simulink model "mppt_top"  (R2025b)
settings: Solver=FixedStepAuto  StartTime=0.0  StopTime=0.05  RelTol=1e-3
PreLoadFcn:
  | addpath('C:\Users\PRANAV\Downloads\ResearchWorks\hdlimport\mppt_top');
libraries: fl_lib x10, simulink x9, nesl_utility x6, hdlsllib x4, ee_lib x1
CloseFcn:
  | addpath('C:\Users\PRANAV\Downloads\ResearchWorks\hdlimport\mppt_top');
  | rmpath('C:\Users\PRANAV\Downloads\ResearchWorks\hdlimport\mppt_top');
settings Model: DataTypeOverride=Off  Creator=PRANAV  LastModifiedBy=PRANAV
settings OptimizationCC: BlockReduction=off  ConditionallyExecuteInputs=off  DefaultParameterBehavior=Inlined  InheritOutputTypeSmallerThanSingle=on
settings DebuggingCC: ArtificialAlgebraicLoopMsg=error  InheritedTsInSrcMsg=none  SingleTaskRateTransMsg=error
settings HardwareCC: ProdBitPerPointer=32.0  ProdBitPerSizeT=32.0  ProdBitPerPtrDiffT=32.0  ProdLargestAtomicFloat=None  ProdIntDivRoundTo=Undefined  ProdEndianess=Unspecified  ProdWordSize=32.0  ProdHWDeviceType=ASIC/FPGA->ASIC/FPGA  TargetBitPerPointer=64.0  TargetBitPerSizeT=64.0  TargetBitPerPtrDiffT=64.0  TargetLongLongMode=on  TargetIntDivRoundTo=Zero  TargetEndianess=LittleEndian  TargetWordSize=64.0  TargetHWDeviceType=Custom Processor->MATLAB Host Computer  ProdEqTarget=off

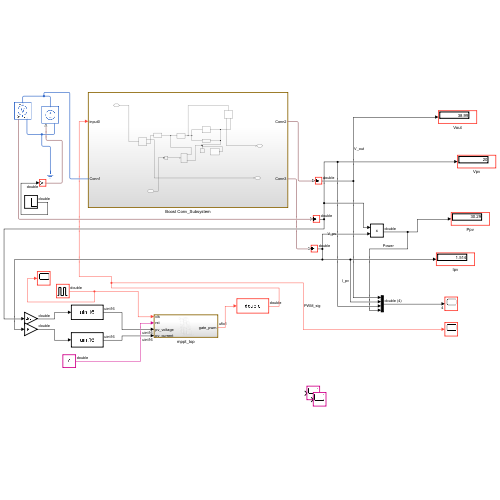
[thumbnail: Simulink's stored preview of the top-level diagram]
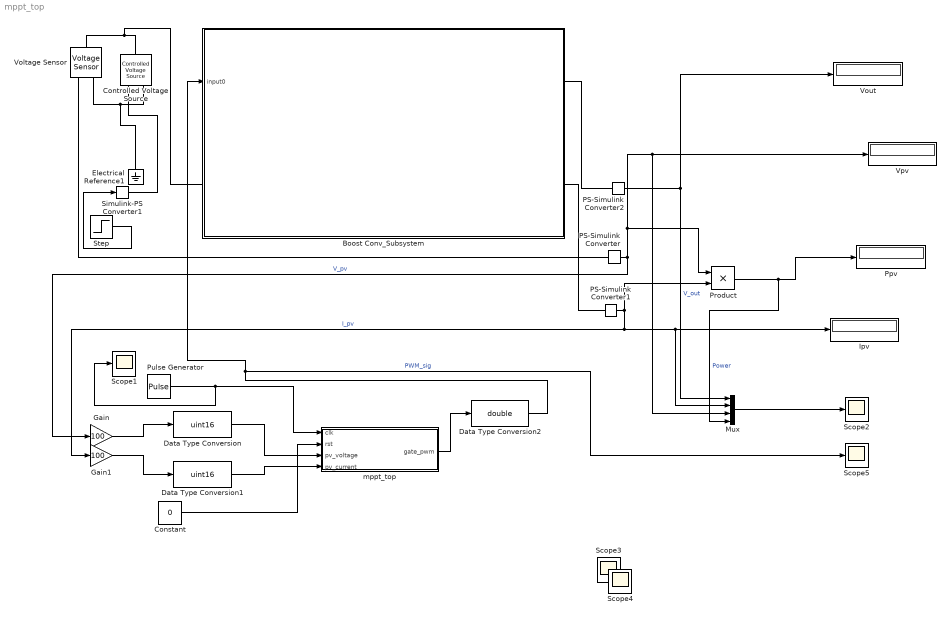
== system mppt_top ==
  Boost Conv_Subsystem : Subsystem
  Constant : Constant  Value=0
  Controlled Voltage Source : fl_lib/Electrical/Electrical Sources/Controlled Voltage Source
  Data Type Conversion : DataTypeConversion  OutDataTypeStr=uint16  SaturateOnIntegerOverflow=off  RndMeth=Floor
  Data Type Conversion1 : DataTypeConversion  OutDataTypeStr=uint16  SaturateOnIntegerOverflow=off  RndMeth=Floor
  Data Type Conversion2 : DataTypeConversion  OutDataTypeStr=double  SaturateOnIntegerOverflow=off  RndMeth=Floor
  Electrical Reference1 : fl_lib/Electrical/Electrical Elements/Electrical Reference
  Gain : Gain  Gain=100
  Gain1 : Gain  Gain=100
  Ipv : Display
  Mux : Mux
  PS-Simulink Converter : nesl_utility/PS-Simulink Converter  PhysicalDomain=network_engine_domain  SubClassName=ps_output  LeftPortType=input  RightPortType=output  PseudoPeriodic=off  Frequencies=[]  VectorFormat=inherit  Unit=inherit  AffineConversion=off
  PS-Simulink Converter1 : nesl_utility/PS-Simulink Converter  PhysicalDomain=network_engine_domain  SubClassName=ps_output  LeftPortType=input  RightPortType=output  PseudoPeriodic=off  Frequencies=[]  VectorFormat=inherit  Unit=inherit  AffineConversion=off
  PS-Simulink Converter2 : nesl_utility/PS-Simulink Converter  PhysicalDomain=network_engine_domain  SubClassName=ps_output  LeftPortType=input  RightPortType=output  PseudoPeriodic=off  Frequencies=[]  VectorFormat=inherit  Unit=inherit  AffineConversion=off
  Ppv : Display
  Product : Product
  Pulse Generator : DiscretePulseGenerator  PulseType=Time based  Period=1e-7  PulseWidth=50
  Scope{1..5} (5 alike) : Scope
      Scope1 settings: ActiveDisplayYMinimum=-0.12499999999999997  ActiveDisplayYMaximum=1.125
      Scope2 settings: ActiveDisplayYMinimum=-1.6786865091982826  ActiveDisplayYMaximum=12.282327357621083  DataLoggingVariableName=ScopeData2
      Scope3 settings: ActiveDisplayYMinimum=-0.35880228687725468  ActiveDisplayYMaximum=10.723962564360617
      Scope4 settings: ActiveDisplayYMinimum=-0.35880228687725468  ActiveDisplayYMaximum=10.723962564360617  DataLoggingVariableName=ScopeData3
      Scope5 settings: ActiveDisplayYMinimum=-0.35880228687725468  ActiveDisplayYMaximum=10.723962564360617  DataLoggingVariableName=ScopeData4
  Simulink-PS Converter1 : nesl_utility/Simulink-PS Converter  PhysicalDomain=network_engine_domain  SubClassName=ps_input  LeftPortType=input  RightPortType=output  PseudoPeriodic=off  Frequencies=[]  NoiseDistribution=none  NoiseParameters=[]  Unit=1  AffineConversion=off  FilteringAndDerivatives=provide  SimscapeFilterOrder=1  InputFilterTimeConstant=0.001  UdotUserProvided=0
  Step : Step  Time=0.2  Before=20  After=15  SampleTime=0
  Voltage Sensor : fl_lib/Electrical/Electrical Sensors/Voltage Sensor
  Vout : Display
  Vpv : Display
  mppt_top : Subsystem
  wires:
  Data Type Conversion/1 -> mppt_top/3(pv_voltage)
  Data Type Conversion1/1 -> mppt_top/4(pv_current)
  PS-Simulink Converter2/1 -> Vout/1, Mux/1  "V_out"
  PS-Simulink Converter1/1 -> Ipv/1, Mux/2, Gain1/1, Product/2  "I_pv"
  PS-Simulink Converter/1 -> Product/1, Vpv/1, Mux/3, Gain/1  "V_pv"
  Product/1 -> Mux/4, Ppv/1  "Power"
  Gain/1 -> Data Type Conversion/1
  Gain1/1 -> Data Type Conversion1/1
  Pulse Generator/1 -> Scope1/1, mppt_top/1(clk)
  Constant/1 -> mppt_top/2(rst)
  mppt_top/1(gate_pwm) -> Data Type Conversion2/1
  Data Type Conversion2/1 -> Boost Conv_Subsystem/1(input0), Scope5/1  "PWM_sig"
  Step/1 -> Simulink-PS Converter1/1
  Mux/1 -> Scope2/1
  connections:
  Electrical Reference1/LConn1 -- Controlled Voltage Source/RConn2 -- Voltage Sensor/RConn2
  Voltage Sensor/LConn1 -- Boost Conv_Subsystem/LConn1 -- Controlled Voltage Source/LConn1
  Voltage Sensor/RConn1 -- PS-Simulink Converter/LConn1
  Simulink-PS Converter1/RConn1 -- Controlled Voltage Source/RConn1
  Boost Conv_Subsystem/RConn1 -- PS-Simulink Converter2/LConn1
  Boost Conv_Subsystem/RConn2 -- PS-Simulink Converter1/LConn1

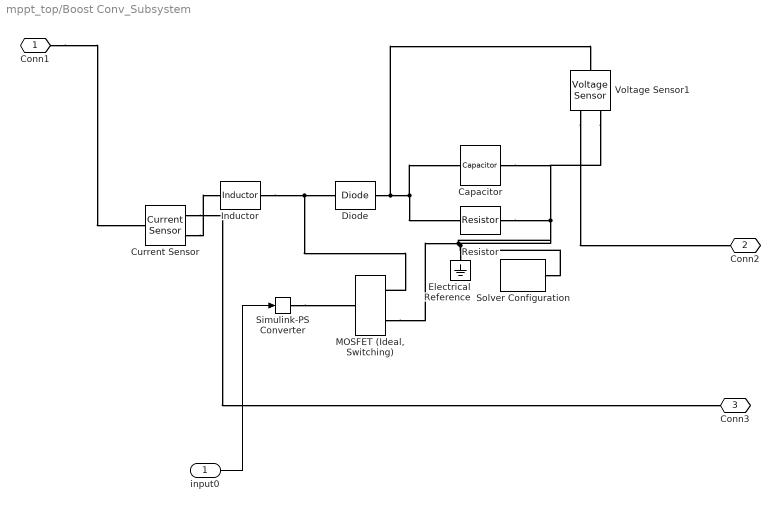
== system mppt_top/Boost Conv_Subsystem ==
  input0 : Inport
  Capacitor : fl_lib/Electrical/Electrical Elements/Capacitor  c=470 uF  r=1e-6 Ohm  g=0 1/Ohm  i_specify=off  i_priority=None  i=0 A  i_nominal_specify=off  i_nominal_value=1  i_nominal_unit=A  v_specify=off  v_priority=None  v=0 V  v_nominal_specify=off  v_nominal_value=1  v_nominal_unit=V  vc_specify=off  vc_priority=High  vc=0 V  vc_nominal_specify=off  vc_nominal_value=1  vc_nominal_unit=V
  Current Sensor : fl_lib/Electrical/Electrical Sensors/Current Sensor
  Diode : fl_lib/Electrical/Electrical Elements/Diode  Vf=0.6 V  Ron=0.3 Ohm  Goff=1e-8 1/Ohm  i_specify=off  i_priority=None  i=0 A  i_nominal_specify=off  i_nominal_value=1  i_nominal_unit=A  v_specify=off  v_priority=None  v=0 V  v_nominal_specify=off  v_nominal_value=1  v_nominal_unit=V
  Electrical Reference : fl_lib/Electrical/Electrical Elements/Electrical Reference
  Inductor : fl_lib/Electrical/Electrical Elements/Inductor  l=1 mH  r=0 Ohm  g=1e-9 1/Ohm  i_specify=off  i_priority=None  i=0 A  i_nominal_specify=off  i_nominal_value=1  i_nominal_unit=A  v_specify=off  v_priority=None  v=0 V  v_nominal_specify=off  v_nominal_value=1  v_nominal_unit=V  i_L_specify=off  i_L_priority=High  i_L=0 A  i_L_nominal_specify=off  i_L_nominal_value=1  i_L_nominal_unit=A
  "MOSFET (Ideal, Switching)" : ee_lib/Semiconductors & Converters/MOSFET (Ideal, Switching)  port_option=ee.enum.controlport.ps  Rds=1e-3 Ohm  Goff=1e-6 1/Ohm  Vth=0.5 V  diode_param=ee.enum.semiconductors.protectionDiode.nodynamics  diode_Vf=0.8 V  diode_Ron=0.001 Ohm  diode_Goff=1e-5 1/Ohm  diode_C=50e-9 F  diode_iRM=-235 A  diode_iF=300 A  diode_idot=-50 A/us  diode_trr_param=ee.enum.converters.diodeReverseParam.trr_factor  diode_trr_factor=3  diode_trr=15 us  diode_Qrr=1500 s*uA  ids_specify=off  ids_priority=None  ids=0 A  ids_nominal_specify=off  ids_nominal_value=1  ids_nominal_unit=A  vds_specify=off  vds_priority=None  vds=0 V  vds_nominal_specify=off  vds_nominal_value=1  vds_nominal_unit=V  vgs_specify=off  vgs_priority=None  vgs=0 V  vgs_nominal_specify=off  vgs_nominal_value=1  vgs_nominal_unit=V  thermal_loss_option=ee.enum.converters.thermalLossOption.constantvalues  Von_data=[0, 1.8, 3.2, 6, 10, 16; 0, 2, 5.5, 9.5, 15, 25] V  Tj=[298.15, 448.15] K  Iout_data=[0, 20, 40, 60, 80, 100] A  Eon_data=[0, 55.04, 124.57, 235.53, 362.12; 0, 71.25, 161.25, 304.88, 468.75] * 1e-6 J  Eoff_data=[0, 18, 30, 56.1, 76.5; 0, 22.5, 37.5, 70.13, 95.63] * 1e-6 J  Eon_data_3D=[zeros(2, 5, 3)] J  Eoff_data_3D=[zeros(2, 5, 3)] J  Tj_loss=[298.15, 448.15] K  Iout_data_loss=[0, 10, 20, 30, 40] A  tabulateWithVds=false  Vds_loss=[0, 150, 300] V  Eon_scalar=22.86e-3 J  Eoff_scalar=17.14e-3 J  Voff=300 V  Iout_scalar=600 A  useCurrentFromPreviousCycle=false  useVoltageFromPreviousCycle=false  diodeModelType=ee.enum.converters.diodeModelType.pwl  diodeTableType=ee.enum.diode.tableType.IfMat  diode_ReverseIVType=ee.enum.diode.diodeReverseIV.constant  diode_IfMat=[.07, .12, .19, 1.75, 4.24, 7.32, 11.2; .16, .3, .72, 2.14, 4.02, 6.35, 9.12] A  diode_VfMat=[.9, 1.15, 1.25, 1.5, 1.75, 2.17, 2.6, 2.85; .58, .68, .75, 1.1, 1.38, 1.77, 2.27, 2.7] V  diode_TjVec=[25, 125] degC  diode_VfVec=[.5, .7, .9, 1.3, 1.7, 2.1, 2.5] V  diode_IfVec=[.1, .2, .5, 1, 2, 4, 7, 10] A  diode_IrMat=[1e-06, 2e-06, 5e-06, 1e-05, 2.5e-05, 5e-05, .0001; 2e-06, 5e-06, 1e-05, 4e-05, 8e-05, .0002, .0005] A  diode_VrMat=[10, 100, 200, 250, 300, 325, 350; 10, 70, 160, 220, 270, 300, 320] V  diode_VrVec=[10, 20, 40, 50, 70, 80, 100] V  diode_IrVec=[1e-06, 2e-06, 5e-06, 1e-05, 2e-05, 5e-05, .0001] A  diode_Vr=-600 V  diode_Ls=150 nH  diode_Erec=0.03 J  diode_rec_loss_model=ee.enum.diode.reverseRecoveryModel.fixed  diode_ErecVal=0 J  diode_scaleWithIandV=true  diode_ErecMat=zeros(2, 3) J  diode_TjrecVec=[298.15, 398.15] K  diode_IfrecVec=[.1, 1, 10] A  diode_IrecVal=10 A  diode_VrecVal=10 V  diode_tFilter=1 / 1000 / 100 s  separateThermalPortForDiode=false  thermal_network_parameterization=ee.enum.thermalNetworkTopology.external  Rth=[.03, .2] K/W  Rth_Cauer=[.03, .1, .2] K/W  Rth_Foster=[.08, .14, .22, .16] K/W  thermal_mass_parameterization=ee.enum.thermalNetwork.timeconstant  thermal_mass=[3, 25] J/K  thermal_mass_Cauer=[3, 10, 25] J/K  thermal_mass_Foster=[.001, .005, .05, .5] J/K  thermal_time_constant=[.1, 5] s  thermal_time_constant_Cauer=[.1, 1, 5] s  thermal_time_constant_Foster=[7e-05, .0007, .01, .08] s  thermal_mass_initial_temperatures=[25, 25] degC  thermal_mass_initial_temperatures_Cauer=[25, 25, 25] degC  junction_thermal_mass=0.1 J/K  Tvec_initial_Foster=[25, 25, 25, 25] degC  RthDiode=[.03, .2] K/W  RthCauerDiode=[.03, .1, .2] K/W  RthFosterDiode=[.03, .2] K/W  thermalMassDiode=[3, 25] J/K  thermalMassCauerDiode=[3, 10, 25] J/K  thermalMassFosterDiode=[33, 50] J/K  thermalTauDiode=[.1, 5] s  thermalTauCauerDiode=[.1, 1, 5] s  thermalTauFosterDiode=[1, 10] s  thermalMassInitTempDiode=[25, 25] degC  thermalMassInitTempCauerDiode=[25, 25, 25] degC  junctionthermalMassDiode=0.1 J/K  TVecInitialFosterDiode=[25, 25, 25, 25] degC  no_thermal_network=0  mosfet_junction_temperature_specify=off  mosfet_junction_temperature_priority=None  mosfet_junction_temperature=25 degC  mosfet_junction_temperature_nominal_specify=off  mosfet_junction_temperature_nominal_value=1  mosfet_junction_temperature_nominal_unit=degC  diode_junction_temperature_specify=off  diode_junction_temperature_priority=None  diode_junction_temperature=25 degC  diode_junction_temperature_nominal_specify=off  diode_junction_temperature_nominal_value=1  diode_junction_temperature_nominal_unit=degC  Qj_specify=off  Qj_priority=None  Qj=0 W  Qj_nominal_specify=off  Qj_nominal_value=1  Qj_nominal_unit=W  accumulatedSwitchingLosses_specify=off  accumulatedSwitchingLosses_priority=None  accumulatedSwitchingLosses=0 J
  Resistor : fl_lib/Electrical/Electrical Elements/Resistor  R=50 Ohm  i_specify=off  i_priority=None  i=0 A  i_nominal_specify=off  i_nominal_value=1  i_nominal_unit=A  v_specify=off  v_priority=None  v=0 V  v_nominal_specify=off  v_nominal_value=1  v_nominal_unit=V
  Simulink-PS Converter : nesl_utility/Simulink-PS Converter  PhysicalDomain=network_engine_domain  SubClassName=ps_input  LeftPortType=input  RightPortType=output  PseudoPeriodic=off  Frequencies=[]  NoiseDistribution=none  NoiseParameters=[]  Unit=1  AffineConversion=off  FilteringAndDerivatives=provide  SimscapeFilterOrder=1  InputFilterTimeConstant=0.001  UdotUserProvided=0
  Solver Configuration : nesl_utility/Solver Configuration  PhysicalDomain=network_engine_domain  SubClassName=solver  LeftPortType=input  RightPortType=generic  Tones=[]  Harmonics=[]  SimulateNoise=off  Profile=off  UseLocalSampling=off  EnableSwitchedLinearOptims=on  FrequencyDomain=off  UseCCode=off  RelTol=0.001  AbsTol=0.001  MinStep=1e-09  ToWorkspace=off  RevertToSquareIcSolve=off  NumHomotopyIterations=100  PhasorMode=off  PhasorModeNumHarmonics=1  ConsistencySolver=NEWTON_XTOL_AFTER_FTOL  IndexReductionMethod=DerivativeReplacement  DoDC=off  ResidualTolerance=1e-09  ConsistencyTolSource=GLOBAL  ConsistencyAbsTol=0.001  ConsistencyRelTol=0.001  ConsistencyTolFactor=0.001  UseLocalSolver=off  LocalSolverChoice=NE_BACKWARD_EULER_ADVANCER  ResolveIndetEquations=on  FunctionEvalNumThread=1  LocalSolverSampleTime=0.001  DoFixedCost=off  MaxNonlinIter=3  MaxModeIter=2  ComputeImpulses=off  ImpulseIterations=2  LinearAlgebra=auto  LinearAlgebraNumThread=0  EquationFormulation=NE_TIME_EF  DelaysMemoryBudget=1024  AutomaticFiltering=on  FilteringTimeConstant=0.001  PartitionStorageMethod=AS_NEEDED  PartitionMemoryBudget=1024  PartitionMethod=ROBUST  MultibodyUseLocalSolver=off  MultibodyLocalSolverChoice=ODE1  MultibodyLocalSolverSampleTime=0.001
  Voltage Sensor1 : fl_lib/Electrical/Electrical Sensors/Voltage Sensor
  Conn1 : PMIOPort  Side=Left
  Conn2 : PMIOPort  Port=2  Side=Right
  Conn3 : PMIOPort  Port=3  Side=Right
  wires:
  input0/1 -> Simulink-PS Converter/1
  connections:
  Conn1/RConn1 -- Current Sensor/LConn1
  Diode/RConn1 -- Voltage Sensor1/LConn1 -- Capacitor/LConn1 -- Resistor/LConn1
  Voltage Sensor1/RConn1 -- Conn2/RConn1
  Inductor/RConn1 -- "MOSFET (Ideal, Switching)"/RConn1 -- Diode/LConn1
  Electrical Reference/LConn1 -- Solver Configuration/RConn1 -- Capacitor/RConn1 -- Voltage Sensor1/RConn2 -- Resistor/RConn1 -- "MOSFET (Ideal, Switching)"/RConn2
  Current Sensor/RConn2 -- Inductor/LConn1
  Simulink-PS Converter/RConn1 -- "MOSFET (Ideal, Switching)"/LConn1
  Current Sensor/RConn1 -- Conn3/RConn1

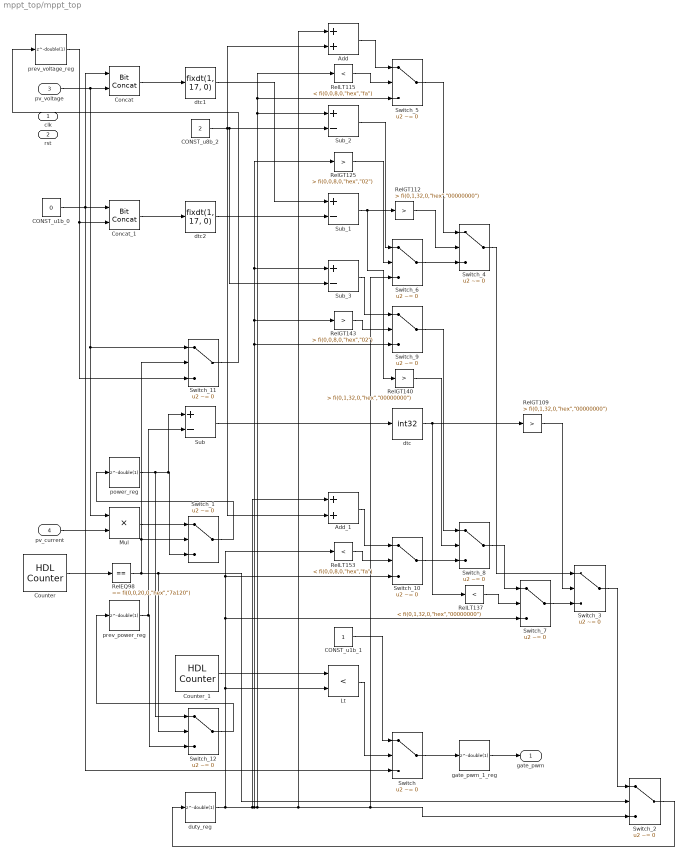
== system mppt_top/mppt_top ==
  clk : Inport
  rst : Inport  Port=2
  pv_voltage : Inport  Port=3  OutDataTypeStr=uint16  SampleTime=-1
  pv_current : Inport  Port=4  OutDataTypeStr=uint16  SampleTime=-1
  Add : Sum  OutDataTypeStr=uint8  AccumDataTypeStr=uint8  SampleTime=-1
  Add_1 : Sum  OutDataTypeStr=uint8  AccumDataTypeStr=uint8  SampleTime=-1
  CONST_u1b_0 : Constant  Value=0  OutDataTypeStr=fixdt(0, 1, 0)  SampleTime=-1
  CONST_u1b_1 : Constant  OutDataTypeStr=fixdt(0, 1, 0)  SampleTime=-1
  CONST_u8b_2 : Constant  Value=2  OutDataTypeStr=uint8  SampleTime=-1
  Concat : hdlsllib/Logic and Bit Operations/Bit Concat  numInputs=2
  Concat_1 : hdlsllib/Logic and Bit Operations/Bit Concat  numInputs=2
  Counter : hdlsllib/Sources/HDL Counter  CountType=Count limited  CountInit="fi(0,0,20,0,\"hex\",\"00000\")"  CountStep="fi(0,0,20,0,\"hex\",\"00001\")"  CountMax="fi(0,0,20,0,\"hex\",\"7a120\")"  CountFromType=Initial value  CountFrom="fi(0,0,20,0,\"hex\",\"00000\")"  CountResetPort=off  CountLoadPort=off  CountEnbPort=off  CountDirPort=off  CountHitOutputPort=off  CountDataType=Unsigned  CountWordLen=20  CountFracLen=0  CountSampTime=-1
  Counter_1 : hdlsllib/Sources/HDL Counter  CountType=Free running  CountInit="fi(0,0,8,0,\"hex\",\"00\")"  CountStep="fi(0,0,8,0,\"hex\",\"01\")"  CountMax="fi(0,0,8,0,\"hex\",\"00\")"  CountFromType=Initial value  CountFrom="fi(0,0,8,0,\"hex\",\"00\")"  CountResetPort=off  CountLoadPort=off  CountEnbPort=off  CountDirPort=off  CountHitOutputPort=off  CountDataType=Unsigned  CountWordLen=8  CountFracLen=0  CountSampTime=-1
  Lt : RelationalOperator  Operator=<  OutDataTypeStr=fixdt(0,1,0)  SampleTime=-1  InputSameDT=off
  Mul : Product  Inputs=**  OutDataTypeStr=uint32  SampleTime=-1
  RelEQ98 : simulink/Logic and Bit Operations/Compare To Constant  relop===  const="fi(0,0,20,0,\"hex\",\"7a120\")"  OutDataTypeStr=boolean
  RelGT109 : simulink/Logic and Bit Operations/Compare To Constant  relop=>  const="fi(0,1,32,0,\"hex\",\"00000000\")"  OutDataTypeStr=boolean
  RelGT112 : simulink/Logic and Bit Operations/Compare To Constant  relop=>  const="fi(0,1,32,0,\"hex\",\"00000000\")"  OutDataTypeStr=boolean
  RelGT125 : simulink/Logic and Bit Operations/Compare To Constant  relop=>  const="fi(0,0,8,0,\"hex\",\"02\")"  OutDataTypeStr=boolean
  RelGT140 : simulink/Logic and Bit Operations/Compare To Constant  relop=>  const="fi(0,1,32,0,\"hex\",\"00000000\")"  OutDataTypeStr=boolean
  RelGT143 : simulink/Logic and Bit Operations/Compare To Constant  relop=>  const="fi(0,0,8,0,\"hex\",\"02\")"  OutDataTypeStr=boolean
  RelLT115 : simulink/Logic and Bit Operations/Compare To Constant  relop=<  const="fi(0,0,8,0,\"hex\",\"fa\")"  OutDataTypeStr=boolean
  RelLT137 : simulink/Logic and Bit Operations/Compare To Constant  relop=<  const="fi(0,1,32,0,\"hex\",\"00000000\")"  OutDataTypeStr=boolean
  RelLT153 : simulink/Logic and Bit Operations/Compare To Constant  relop=<  const="fi(0,0,8,0,\"hex\",\"fa\")"  OutDataTypeStr=boolean
  Sub : Sum  Inputs=+-  OutDataTypeStr=uint32  AccumDataTypeStr=uint32  SampleTime=-1
  Sub_1 : Sum  Inputs=+-  OutDataTypeStr=fixdt(1, 17, 0)  AccumDataTypeStr=fixdt(1, 17, 0)  SampleTime=-1
  Sub_2 : Sum  Inputs=+-  OutDataTypeStr=uint8  AccumDataTypeStr=uint8  SampleTime=-1
  Sub_3 : Sum  Inputs=+-  OutDataTypeStr=uint8  AccumDataTypeStr=uint8  SampleTime=-1
  Switch : Switch  Criteria=u2 ~= 0  Threshold="fi(0,0,1,0,\"hex\",\"0\")"  OutDataTypeStr=fixdt(0, 1, 0)  SampleTime=-1  SaturateOnIntegerOverflow=off  InputSameDT=off
  Switch_1 : Switch  Criteria=u2 ~= 0  Threshold="fi(0,0,1,0,\"hex\",\"0\")"  OutDataTypeStr=uint32  SampleTime=-1  SaturateOnIntegerOverflow=off  InputSameDT=off
  Switch_{2..10} (9 alike) : Switch  Criteria=u2 ~= 0  Threshold="fi(0,0,1,0,\"hex\",\"0\")"  OutDataTypeStr=uint8  SampleTime=-1  SaturateOnIntegerOverflow=off  InputSameDT=off
  Switch_11 : Switch  Criteria=u2 ~= 0  Threshold="fi(0,0,1,0,\"hex\",\"0\")"  OutDataTypeStr=uint16  SampleTime=-1  SaturateOnIntegerOverflow=off  InputSameDT=off
  Switch_12 : Switch  Criteria=u2 ~= 0  Threshold="fi(0,0,1,0,\"hex\",\"0\")"  OutDataTypeStr=uint32  SampleTime=-1  SaturateOnIntegerOverflow=off  InputSameDT=off
  dtc : DataTypeConversion  OutDataTypeStr=int32  SampleTime=-1  SaturateOnIntegerOverflow=off  RndMeth=Floor
  dtc1 : DataTypeConversion  OutDataTypeStr=fixdt(1, 17, 0)  SampleTime=-1  SaturateOnIntegerOverflow=off  RndMeth=Floor
  dtc2 : DataTypeConversion  OutDataTypeStr=fixdt(1, 17, 0)  SampleTime=-1  SaturateOnIntegerOverflow=off  RndMeth=Floor
  duty_reg : Delay  DelayLength=double(1)  InitialCondition=128  SampleTime=-1
  gate_pwm_1_reg : Delay  DelayLength=double(1)  InitialCondition=0  SampleTime=-1
  power_reg : Delay  DelayLength=double(1)  InitialCondition=0  SampleTime=-1
  prev_power_reg : Delay  DelayLength=double(1)  InitialCondition=0  SampleTime=-1
  prev_voltage_reg : Delay  DelayLength=double(1)  InitialCondition=0  SampleTime=-1
  gate_pwm : Outport  OutDataTypeStr=fixdt(0, 1, 0)  SampleTime=-1
  wires:
  prev_voltage_reg/1 -> Switch_11/3, Concat_1/2
  pv_voltage/1 -> Mul/1, Switch_11/1, Concat/2
  Concat_1/1 -> dtc2/1
  CONST_u1b_0/1 -> Switch/3, Concat_1/1, Concat/1
  pv_current/1 -> Mul/2
  Add_1/1 -> Switch_10/1
  Counter/1 -> RelEQ98/1
  Concat/1 -> dtc1/1
  power_reg/1 -> Switch_1/3, Sub/1, Switch_12/1
  Sub_1/1 -> RelGT140/1, RelGT112/1
  Mul/1 -> Switch_1/1
  RelEQ98/1 -> Switch_12/2, Switch_2/2, Switch_11/2, Switch_1/2
  Switch_10/1 -> Switch_8/3
  prev_power_reg/1 -> Switch_12/3, Sub/2
  Lt/1 -> Switch/2
  dtc1/1 -> Sub_1/1
  CONST_u8b_2/1 -> Sub_2/2, Sub_3/2, Add/2, Add_1/2
  RelLT137/1 -> Switch_7/2
  dtc2/1 -> Sub_1/2
  RelLT115/1 -> Switch_5/2
  Switch_11/1 -> prev_voltage_reg/1
  Sub/1 -> dtc/1
  Switch_1/1 -> power_reg/1
  Counter_1/1 -> Lt/1
  Add/1 -> Switch_5/1
  Switch_12/1 -> prev_power_reg/1
  duty_reg/1 -> Switch_2/3, Switch_6/3, Add/1, Switch_5/3, RelLT115/1, Sub_2/1, Sub_3/1, RelGT125/1, RelGT143/1, Switch_9/3, Add_1/1, Switch_10/3, RelLT153/1, Switch_7/3, Lt/2
  Sub_2/1 -> Switch_6/1
  RelGT125/1 -> Switch_6/2
  Sub_3/1 -> Switch_9/1
  RelGT143/1 -> Switch_9/2
  RelLT153/1 -> Switch_10/2
  CONST_u1b_1/1 -> Switch/1
  Switch_5/1 -> Switch_4/1
  RelGT112/1 -> Switch_4/2
  Switch_6/1 -> Switch_4/3
  Switch_9/1 -> Switch_8/1
  RelGT140/1 -> Switch_8/2
  dtc/1 -> RelGT109/1, RelLT137/1
  Switch/1 -> gate_pwm_1_reg/1
  Switch_4/1 -> Switch_3/1
  Switch_8/1 -> Switch_7/1
  gate_pwm_1_reg/1 -> gate_pwm/1
  RelGT109/1 -> Switch_3/2
  Switch_7/1 -> Switch_3/3
  Switch_3/1 -> Switch_2/1
  Switch_2/1 -> duty_reg/1
